simulink model "sm_boom_lift_crawler_test_jib_hydr_3D"  (R2026a)
settings: Solver=ode23t  StopTime=tVec.StopTime  MaxStep=2  AbsTol=1e-3
PostLoadFcn:
  | sm_boom_lift_crawler_settest('jib test')
StartFcn:
  | tic;
StopFcn:
  | Elapsed_Sim_Time = toc;
  | %disp(['Elapsed Sim Time = ' num2str(Elapsed_Sim_Time)]);
undefined symbols (not defined in the file): motion, oVec, tVec, X, Y, Z
libraries: nesl_utility x5, sm_lib x5, sm_boom_lift_crawler_lib x4, fl_lib x2, sm_boom_lift_crawler_lib_boom x1, sm_boom_lift_crawler_lib_actuators x1, sm_boom_lift_crawler_lib_inputs x1, simulink_extras x1
Description:
  | Copyright 2025-2026 The MathWorks, Inc.
settings Model: Creator=smiller  LastModifiedBy=smiller
settings SolverCC: MaxConsecutiveMinStep=5
settings DataIOCC: SignalLoggingName=logsout_sm_boom_lift_crawler
settings SimscapeCC: SimscapeNominalValues="[{\"value\":\"1\",\"unit\":\"A\"},{\"value\":\"nomval_psi\",\"unit\":\"psi\"},{\"value\":\"1\",\"unit\":\"cm^2\"},{\"value\":\"nomval_cmv3_s\",\"unit\":\"cm^3/s\"},{\"value\":\"1\",\"unit\":\"kJ/kg\"},{\"value\":\"1\",\"unit\":\"kW\"},{\"value\":\"1\",\"unit\":\"l\"},{\"value\":\"nomval_N\",\"unit\":\"N\"},{\"value\":\"nomval_Nm\",\"unit\":\"N*m\"},{\"value\":\"1\",\"unit\":\"V\"}]"  SimscapeLogName=simlog_sm_boom_lift_crawler  SimscapeLogLimitData=off  SimscapeLogDataHistory=5000.0
settings DiagnosticsConfigSet: SimMechanicsConflictingReferenceFrames=none  SimMechanicsRigidlyBoundBlock=none
settings ExplorerConfigSet: InternalSimMechanicsExplorerSettings="<ExplorerConfiguration><canonicalview>default</canonicalview><AnimationSetting><BasePlaybackSpeed>1.0</BasePlaybackSpeed><PlaybackSpeedFactor>8.0</PlaybackSpeedFactor></AnimationSetting><TilePanel><TileInfo><Tiles Columns=\"1\" Count=\"1\" Rows=\"1\"><Column Weight=\"1\"/><Row Weight=\"1\"/><Tile Height=\"1\" Width=\"1\" X=\"0\" Y=\"0\"/></Tiles></TileInfo><SceneInfo><SceneViewer><BGColor><R>1</R><G>1</G><B>1</B></BGColor><Camera><DoPerspective>on</DoPerspective><Position><X>3</X><Y>-0.999366517742438232</Y><Z>-0.50126496308374946</Z></Position><Center><X>2</X><Y>-0.999366517742438343</Y><Z>-0.501264963083749349</Z></Center><Up><X>0</X><Y>0</Y><Z>1</Z></Up><ViewLimDist>1</ViewLimDist><YLim>0.466307658154998583</YLim><XLim>0.785360266366313398</XLim></Camera></SceneViewer></SceneInfo></TilePanel><MechEditorPanel><Cameras><Camera><Id>Camera10</Id><Value><Name>Basket_Rotate</Name><NativeCamera><PositionTrackingFeature>Basket.Basket_Rotate.Bracket.Reference_Camera_Basket_Rotate_L.R</PositionTrackingFeature><CenterTrackingFeature>Basket.Basket_Rotate.Bracket.Reference_Camera_Basket_Rotate_L.R</CenterTrackingFeature><UpVectorTrackingFeature>Basket.Basket_Rotate.Bracket.Reference_Camera_Basket_Rotate_L.R</UpVectorTrackingFeature><CenterTrackingOrigin>off</CenterTrackingOrigin><CenterTrackingDirection>-X</CenterTrackingDirection><UpVectorTrackingDirection>+Z</UpVectorTrackingDirection></NativeCamera></Value></Camera><Camera><Id>Camera13</Id><Value><Name>View_Basket_World</Name><NativeCamera><PositionTrackingFeature>Basket.Basket.Reference_Basket_Cam.R</PositionTrackingFeature><CenterTrackingFeature>Mech_Config.World.W</CenterTrackingFeature><UpVectorTrackingFeature>Basket.Basket.Reference_Basket_Cam.R</UpVectorTrackingFeature><CenterTrackingOrigin>on</CenterTrackingOrigin><UpVectorTrackingDirection>+Y</UpVectorTrackingDirection></NativeCamera></Value></Camera><Camera><Id>Camera17</Id><Value><Name>Jib</Name><NativeCamera><PositionTrackingFeature>Basket.Jib.Jib_Mount.Reference_Camera_Basket_Jib.R</PositionTrackingFeature><CenterTrackingFeature>Basket.Jib.Jib_Mount.Reference_Camera_Basket_Jib.R</CenterTrackingFeature><UpVectorTrackingFeature>Mech_Config.World.W</UpVectorTrackingFeature><CenterTrackingOrigin>off</CenterTrackingOrigin><CenterTrackingDirection>-X</CenterTrackingDirection><UpVectorTrackingDirection>+Z</UpVectorTrackingDirection></NativeCamera></Value></Camera></Cameras><GfxPanelCameraMap><MapElement CameraMLId=\"Camera17\" GfxPanelIndex=\"0\"/></GfxPanelCameraMap><VideoCreator><PlaybackSpeedRatio>8</PlaybackSpeedRatio><FrameRate>30</FrameRate><VideoFormat>MPEG-4</VideoFormat><FrameSize>auto</FrameSize></VideoCreator></MechEditorPanel></ExplorerConfiguration>"

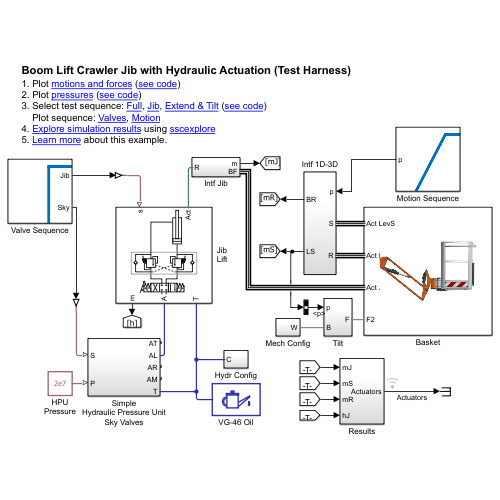
[thumbnail: Simulink's stored preview of the top-level diagram]
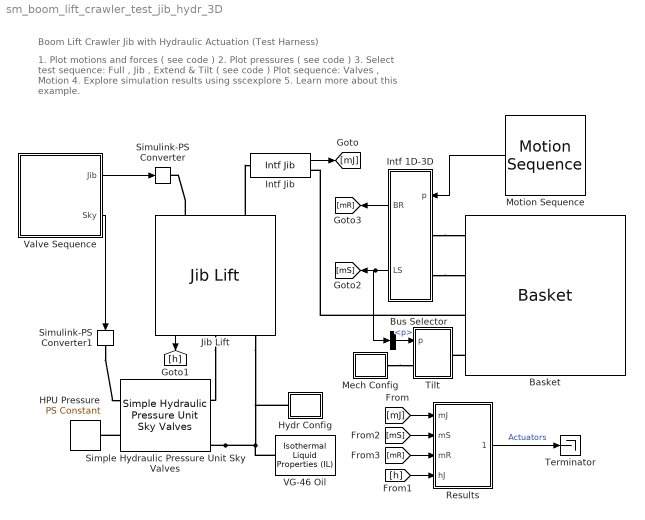
== system sm_boom_lift_crawler_test_jib_hydr_3D ==
  note: 1. Plot motions and forces ( see code )
      | 2. Plot pressures ( see code )
      | 3. Select test sequence: Full , Jib , Extend & Tilt ( see code )
      | Plot sequence: Valves , Motion
      | 4. Explore simulation results using sscexplore
      | 5. Learn more about this example.
  note: Boom Lift Crawler Jib with Hydraulic Actuation (Test Harness)
  Basket : sm_boom_lift_crawler_lib_boom/Boom/Basket  SystemSampleTime=-1  VariantActivationTime=update diagram  EmptyChoice=off  PassThrough=off  PassThroughVariantControl=(default)  EmptyChoiceVariantControl=(default)  AllowFlexibleInterface=on  Latency=0  AutoFrameSizeCalculation=off
  Bus Selector : BusSelector  OutputSignals=p
  HPU Pressure : fl_lib/Physical Signals/Sources/PS Constant  constant=2e7 Pa
  Hydr Config : Subsystem
  Intf 1D-3D : Subsystem
  Intf Jib : sm_boom_lift_crawler_lib/Intf Jib  SystemSampleTime=-1  VariantActivationTime=update diagram  EmptyChoice=off  PassThrough=off  PassThroughVariantControl=(default)  EmptyChoiceVariantControl=(default)  AllowFlexibleInterface=on  Latency=0  AutoFrameSizeCalculation=off
  Jib Lift : sm_boom_lift_crawler_lib_actuators/Actuators/Sky Manifold/Sky Valves II/Jib Lift  SystemSampleTime=-1  VariantActivationTime=update diagram  EmptyChoice=off  PassThrough=off  PassThroughVariantControl=(default)  EmptyChoiceVariantControl=(default)  AllowFlexibleInterface=on  Latency=0  AutoFrameSizeCalculation=off
  Mech Config : Subsystem
  Motion Sequence : sm_boom_lift_crawler_lib_inputs/Motion Sequence  SystemSampleTime=-1  VariantActivationTime=update diagram  EmptyChoice=off  PassThrough=off  PassThroughVariantControl=(default)  EmptyChoiceVariantControl=(default)  AllowFlexibleInterface=on  Latency=0  AutoFrameSizeCalculation=off
  Results : Subsystem
  Simple Hydraulic Pressure Unit Sky Valves : sm_boom_lift_crawler_lib/Simple Hydraulic Pressure Unit Sky Valves  SystemSampleTime=-1  VariantActivationTime=update diagram  EmptyChoice=off  PassThrough=off  PassThroughVariantControl=(default)  EmptyChoiceVariantControl=(default)  AllowFlexibleInterface=on  Latency=0  AutoFrameSizeCalculation=off
  Simulink-PS Converter : nesl_utility/Simulink-PS Converter  PhysicalDomain=network_engine_domain  SubClassName=ps_input  LeftPortType=input  RightPortType=output  PseudoPeriodic=off  Frequencies=[]  NoiseDistribution=none  NoiseParameters=[]  Unit=1  AffineConversion=off  FilteringAndDerivatives=provide  SimscapeFilterOrder=1  InputFilterTimeConstant=0.001  UdotUserProvided=0
  Simulink-PS Converter1 : nesl_utility/Simulink-PS Converter  PhysicalDomain=network_engine_domain  SubClassName=ps_input  LeftPortType=input  RightPortType=output  PseudoPeriodic=off  Frequencies=[]  NoiseDistribution=none  NoiseParameters=[]  Unit=1  AffineConversion=off  FilteringAndDerivatives=provide  SimscapeFilterOrder=1  InputFilterTimeConstant=0.001  UdotUserProvided=0
  Terminator : Terminator
  Tilt : Subsystem
  VG-46 Oil : fl_lib/Isothermal Liquid/Utilities/Isothermal Liquid Properties (IL)  rho_L_atm=867.346 kg/m^3  bulk_modulus_model=foundation.enum.bulk_modulus_model.const  beta_gain=6  beta_L_atm=1.48150e+09 Pa  nu_atm=(45.7333)*(1) cSt  p_atm=0.101325 MPa  p_min=1 Pa  properties_range_check=simscape.enum.assert.action.error  air_fraction=ratio_dissolved_air  polytropic_index=1.0  rho_g_atm=1.225 kg/m^3  air_dissolution_model=simscape.enum.onoff.off  p_crit=3 MPa
  Valve Sequence : Subsystem
      mask Display: image('sm_boom_lift_crawler_valve_seq_outputonly.svg');
  wires:
  Motion Sequence/1 -> Intf 1D-3D/1(p)
  Valve Sequence/2(Sky) -> Simulink-PS Converter1/1
  Intf 1D-3D/1(BR) -> [mR]
  [mR] -> Results/3(mR)
  Bus Selector/1 -> Tilt/1(p)  "<p>"
  [h] -> Results/4(hJ)
  Intf 1D-3D/2(LS) -> Bus Selector/1, [mS]
  Results/1(Actuators) -> Terminator/1  "Actuators"
  [mJ] -> Results/1(mJ)
  [mS] -> Results/2(mS)
  Intf Jib/1 -> [mJ]
  Jib Lift/1 -> [h]
  Valve Sequence/1(Jib) -> Simulink-PS Converter/1
  connections:
  Simple Hydraulic Pressure Unit Sky Valves/RConn5 -- Hydr Config/RConn1 -- Jib Lift/RConn2 -- VG-46 Oil/RConn1
  Basket/RConn3 -- Intf Jib/RConn1
  Mech Config/LConn1 -- Tilt/LConn1
  Simulink-PS Converter1/RConn1 -- Simple Hydraulic Pressure Unit Sky Valves/LConn1
  Intf 1D-3D/LConn1 -- Basket/RConn1
  Simple Hydraulic Pressure Unit Sky Valves/LConn2 -- HPU Pressure/RConn1
  Intf 1D-3D/LConn2 -- Basket/RConn2
  Jib Lift/LConn2 -- Intf Jib/LConn1
  Basket/RConn4 -- Tilt/RConn1
  Jib Lift/LConn1 -- Simulink-PS Converter/RConn1
  Jib Lift/RConn1 -- Simple Hydraulic Pressure Unit Sky Valves/RConn2

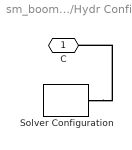
== system sm_boom_lift_crawler_test_jib_hydr_3D/Hydr Config ==
  Solver Configuration : nesl_utility/Solver Configuration  PhysicalDomain=network_engine_domain  SubClassName=solver  LeftPortType=input  RightPortType=generic  Tones=[]  Harmonics=[]  SimulateNoise=off  Profile=off  UseLocalSampling=off  EnableSwitchedLinearOptims=on  FrequencyDomain=off  UseCCode=off  RelTol=0.001  AbsTol=1e-06  MinStep=1e-09  ToWorkspace=off  RevertToSquareIcSolve=off  NumHomotopyIterations=100  PhasorMode=off  PhasorModeNumHarmonics=1  ConsistencySolver=NEWTON_FTOL  CanonicalOrdering=UNORDERED  OptimizeIntermediates=UNOPTIMIZED  IndexReductionMethod=DerivativeReplacement  DoDC=off  ResidualTolerance=1e-9  ConsistencyTolSource=GLOBAL  ConsistencyAbsTol=0.001  ConsistencyRelTol=0.001  ConsistencyTolFactor=0.001  UseLocalSolver=off  LocalSolverChoice=NE_BACKWARD_EULER_ADVANCER  ResolveIndetEquations=on  FunctionEvalNumThread=1  LocalSolverSampleTime=2e-3  DoFixedCost=off  MaxNonlinIter=5  MaxModeIter=2  ComputeImpulses=off  ImpulseIterations=2  LinearAlgebra=Sparse  LinearAlgebraNumThread=0  EquationFormulation=NE_TIME_EF  DelaysMemoryBudget=1024  AutomaticFiltering=on  FilteringTimeConstant=1e-3  PartitionStorageMethod=EXHAUSTIVE  PartitionMemoryBudget=1024  PartitionMethod=FAST  MultibodyUseLocalSolver=off  MultibodyLocalSolverChoice=ODE1  MultibodyLocalSolverSampleTime=0.001
  C : PMIOPort  Side=Right
  connections:
  Solver Configuration/RConn1 -- C/RConn1

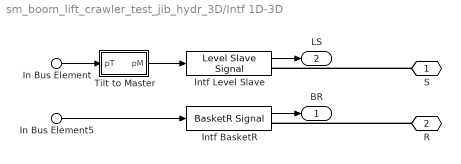
== system sm_boom_lift_crawler_test_jib_hydr_3D/Intf 1D-3D ==
  In Bus Element5 : Inport  PortName=p  Element=BasketR
  In Bus Element : Inport  PortName=p  Element=Tilt
  Intf BasketR : sm_boom_lift_crawler_lib/BasketR Signal  SystemSampleTime=-1  VariantActivationTime=update diagram  EmptyChoice=off  PassThrough=off  PassThroughVariantControl=(default)  EmptyChoiceVariantControl=(default)  AllowFlexibleInterface=on  Latency=0  AutoFrameSizeCalculation=off
  Intf Level Slave : sm_boom_lift_crawler_lib/Level Slave Signal  SystemSampleTime=-1  VariantActivationTime=update diagram  EmptyChoice=off  PassThrough=off  PassThroughVariantControl=(default)  EmptyChoiceVariantControl=(default)  AllowFlexibleInterface=on  Latency=0  AutoFrameSizeCalculation=off
  Tilt to Master : Subsystem
  S : PMIOPort  Side=Left
  R : PMIOPort  Port=2  Side=Left
  BR : Outport
  LS : Outport  Port=2
  wires:
  Intf Level Slave/1 -> LS/1
  Intf BasketR/1 -> BR/1
  In Bus Element5/1 -> Intf BasketR/1
  In Bus Element/1 -> Tilt to Master/1(pT)
  Tilt to Master/1(pM) -> Intf Level Slave/1
  connections:
  S/RConn1 -- Intf Level Slave/RConn1
  R/RConn1 -- Intf BasketR/RConn1

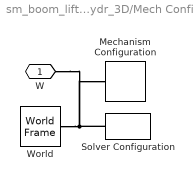
== system sm_boom_lift_crawler_test_jib_hydr_3D/Mech Config ==
  Mechanism Configuration : sm_lib/Utilities/Mechanism Configuration  UniformGravity=Constant  GravityVector=[0 0 -9.80665]  GravityVectorUnits=m/s^2  LinearizationDelta=0.001  JointModeTransitionNonlinearIterations=2
  Solver Configuration : nesl_utility/Solver Configuration  PhysicalDomain=network_engine_domain  SubClassName=solver  LeftPortType=input  RightPortType=generic  Tones=[]  Harmonics=[]  SimulateNoise=off  Profile=off  UseLocalSampling=off  EnableSwitchedLinearOptims=on  FrequencyDomain=off  UseCCode=off  RelTol=0.001  AbsTol=1e-06  MinStep=1e-09  ToWorkspace=off  RevertToSquareIcSolve=off  NumHomotopyIterations=100  PhasorMode=off  PhasorModeNumHarmonics=1  ConsistencySolver=NEWTON_FTOL  CanonicalOrdering=UNORDERED  OptimizeIntermediates=UNOPTIMIZED  IndexReductionMethod=DerivativeReplacement  DoDC=off  ResidualTolerance=1e-9  ConsistencyTolSource=GLOBAL  ConsistencyAbsTol=0.001  ConsistencyRelTol=0.001  ConsistencyTolFactor=0.001  UseLocalSolver=off  LocalSolverChoice=NE_BACKWARD_EULER_ADVANCER  ResolveIndetEquations=on  FunctionEvalNumThread=1  LocalSolverSampleTime=2e-3  DoFixedCost=off  MaxNonlinIter=3  MaxModeIter=2  ComputeImpulses=off  ImpulseIterations=2  LinearAlgebra=auto  LinearAlgebraNumThread=0  EquationFormulation=NE_TIME_EF  DelaysMemoryBudget=1024  AutomaticFiltering=on  FilteringTimeConstant=0.001  PartitionStorageMethod=AS_NEEDED  PartitionMemoryBudget=1024  PartitionMethod=ROBUST  MultibodyUseLocalSolver=off  MultibodyLocalSolverChoice=ODE1  MultibodyLocalSolverSampleTime=0.001
  World : sm_lib/Frames and Transforms/World Frame
  W : PMIOPort  Side=Left
  connections:
  Solver Configuration/RConn1 -- W/RConn1 -- Mechanism Configuration/RConn1 -- World/RConn1

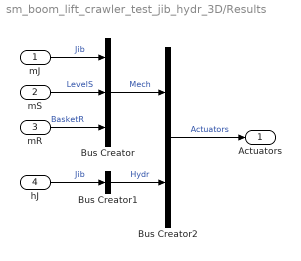
== system sm_boom_lift_crawler_test_jib_hydr_3D/Results ==
  mJ : Inport
  mS : Inport  Port=2
  mR : Inport  Port=3
  hJ : Inport  Port=4
  Bus Creator : BusCreator  Inputs=3
  Bus Creator1 : BusCreator  Inputs=1
  Bus Creator2 : BusCreator  Inputs=2
  Actuators : Outport
  wires:
  Bus Creator/1 -> Bus Creator2/1  "Mech"
  Bus Creator1/1 -> Bus Creator2/2  "Hydr"
  hJ/1 -> Bus Creator1/1  "Jib"
  mJ/1 -> Bus Creator/1  "Jib"
  Bus Creator2/1 -> Actuators/1  "Actuators"
  mS/1 -> Bus Creator/2  "LevelS"
  mR/1 -> Bus Creator/3  "BasketR"

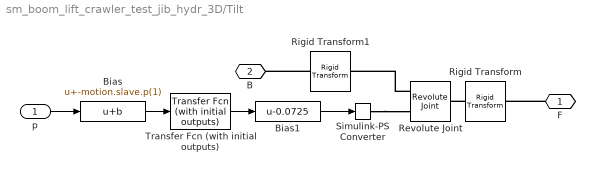
== system sm_boom_lift_crawler_test_jib_hydr_3D/Tilt ==
  p : Inport
  Bias : Bias  Bias=-motion.slave.p(1)  SaturateOnIntegerOverflow=off
  Bias1 : Bias  Bias=-0.0725  SaturateOnIntegerOverflow=off
  Revolute Joint : sm_lib/Joints/Revolute Joint  JointMode=Normal  CompositeWrenchDir=FollowerOnBase  CompositeWrenchFrame=BaseFrame  SenseConstraintForce=off  SenseConstraintTorque=off  SenseTotalForce=off  SenseTotalTorque=off  PositionTargetSpecify=on  PositionTargetPriority=High  PositionTargetValue=-0.0725  PositionTargetValueUnits=deg  VelocityTargetSpecify=off  VelocityTargetPriority=High  VelocityTargetValue=0  VelocityTargetValueUnits=deg/s  EquilibriumPosition=0  EquilibriumPositionUnits=deg  SpringStiffness=0  SpringStiffnessUnits=N*m/deg  DampingCoefficient=0  DampingCoefficientUnits=N*m/(deg/s)  LowerLimitSpecify=off  LowerLimitBound=-90  LowerLimitBoundUnits=deg  LowerLimitStiffness=1e4  LowerLimitStiffnessUnits=N*m/deg  LowerLimitDamping=10  LowerLimitDampingUnits=N*m/(deg/s)  LowerLimitTransitionRegionWidth=0.1  LowerLimitTransitionRegionWidthUnits=deg  UpperLimitSpecify=off  UpperLimitBound=90  UpperLimitBoundUnits=deg  UpperLimitStiffness=1e4  UpperLimitStiffnessUnits=N*m/deg  UpperLimitDamping=10  UpperLimitDampingUnits=N*m/(deg/s)  UpperLimitTransitionRegionWidth=0.1  UpperLimitTransitionRegionWidthUnits=deg  TorqueActuationMode=ComputedTorque  MotionActuationMode=InputMotion  SensePosition=off  SenseVelocity=off  SenseAcceleration=off  SenseTorqueForce=off  SenseLowerLimitTorqueForce=off  SenseUpperLimitTorqueForce=off
  Rigid Transform : sm_lib/Frames and Transforms/Rigid Transform  RotationMethod=StandardAxis  FollAlignAxisA=+X  BaseAlignAxisA=+Y  FollAlignAxisB=+Y  BaseAlignAxisB=+Z  RotationStandardAxis=+Y  RotationAngle=90  RotationAngleUnits=deg  RotationArbitraryAxis=[0 0 1]  RotationSequenceAxes=FollowerAxes  RotationSequence=XYX  RotationSequenceAngles=[0 0 0]  RotationSequenceAnglesUnits=deg  RotationMatrix=[1 0 0; 0 1 0; 0 0 1]  Quaternion=[1 0 0 0]  TranslationMethod=None  TranslationCartesianOffset=[0 0 0]  TranslationCartesianOffsetUnits=m  TranslationStandardAxis=+Z  TranslationStandardOffset=0  TranslationStandardOffsetUnits=m  TranslationROffset=0  TranslationROffsetUnits=m  TranslationThetaOffset=0  TranslationThetaOffsetUnits=deg  TranslationZOffset=0  TranslationZOffsetUnits=m
  Rigid Transform1 : sm_lib/Frames and Transforms/Rigid Transform  RotationMethod=StandardAxis  FollAlignAxisA=+X  BaseAlignAxisA=+Y  FollAlignAxisB=+Y  BaseAlignAxisB=+Z  RotationStandardAxis=+Y  RotationAngle=-90  RotationAngleUnits=deg  RotationArbitraryAxis=[0 0 1]  RotationSequenceAxes=FollowerAxes  RotationSequence=XYX  RotationSequenceAngles=[0 0 0]  RotationSequenceAnglesUnits=deg  RotationMatrix=[1 0 0; 0 1 0; 0 0 1]  Quaternion=[1 0 0 0]  TranslationMethod=None  TranslationCartesianOffset=[0 0 0]  TranslationCartesianOffsetUnits=m  TranslationStandardAxis=+Z  TranslationStandardOffset=0  TranslationStandardOffsetUnits=m  TranslationROffset=0  TranslationROffsetUnits=m  TranslationThetaOffset=0  TranslationThetaOffsetUnits=deg  TranslationZOffset=0  TranslationZOffsetUnits=m
  Simulink-PS Converter : nesl_utility/Simulink-PS Converter  PhysicalDomain=network_engine_domain  SubClassName=ps_input  LeftPortType=input  RightPortType=output  PseudoPeriodic=off  Frequencies=[]  NoiseDistribution=none  NoiseParameters=[]  Unit=deg  AffineConversion=off  FilteringAndDerivatives=filter  SimscapeFilterOrder=2  InputFilterTimeConstant=0.1  UdotUserProvided=0
  Transfer Fcn (with initial outputs) : simulink_extras/Additional Linear/Transfer Fcn (with initial outputs)  N=[400]  D="[0.1  1]"  Y0=0  U0=0
  F : PMIOPort  Side=Right
  B : PMIOPort  Port=2  Side=Left
  wires:
  Transfer Fcn (with initial outputs)/1 -> Bias1/1
  p/1 -> Bias/1
  Bias/1 -> Transfer Fcn (with initial outputs)/1
  Bias1/1 -> Simulink-PS Converter/1
  connections:
  F/RConn1 -- Rigid Transform/RConn1
  Revolute Joint/LConn1 -- Rigid Transform1/RConn1
  Rigid Transform1/LConn1 -- B/RConn1
  Rigid Transform/LConn1 -- Revolute Joint/RConn1
  Simulink-PS Converter/RConn1 -- Revolute Joint/LConn2

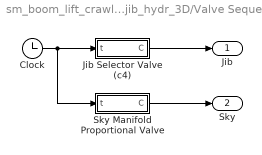
== system sm_boom_lift_crawler_test_jib_hydr_3D/Valve Sequence ==
  Clock : Clock
  Jib Selector Valve (c4) : Subsystem
  Sky Manifold Proportional Valve : Subsystem
  Jib : Outport
  Sky : Outport  Port=2
  wires:
  Sky Manifold Proportional Valve/1(C) -> Sky/1
  Clock/1 -> Jib Selector Valve (c4)/1(t), Sky Manifold Proportional Valve/1(t)
  Jib Selector Valve (c4)/1(C) -> Jib/1

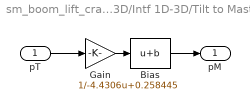
== system sm_boom_lift_crawler_test_jib_hydr_3D/Intf 1D-3D/Tilt to Master ==
  pT : Inport
  Bias : Bias  Bias=0.258445  SaturateOnIntegerOverflow=off
  Gain : Gain  Gain=1/-4.4306
  pM : Outport
  wires:
  Gain/1 -> Bias/1
  pT/1 -> Gain/1
  Bias/1 -> pM/1

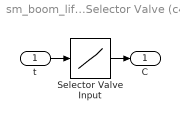
== system sm_boom_lift_crawler_test_jib_hydr_3D/Valve Sequence/Jib Selector Valve (c4) ==
  t : Inport
  Selector Valve Input : Lookup_n-D  NumberOfTableDimensions=1  BreakpointsForDimension1=tVec.sky.c4.all  Table=oVec.sky.c4.all  InterpMethod=Flat  ExtrapMethod=Clip  UseLastTableValue=on  InternalRulePriority=Speed  RndMeth=Simplest
  C : Outport
  wires:
  Selector Valve Input/1 -> C/1
  t/1 -> Selector Valve Input/1

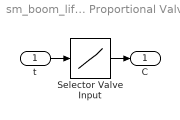
== system sm_boom_lift_crawler_test_jib_hydr_3D/Valve Sequence/Sky Manifold Proportional Valve ==
  t : Inport
  Selector Valve Input : Lookup_n-D  NumberOfTableDimensions=1  BreakpointsForDimension1=tVec.sky.proportional  Table=oVec.sky.proportional  InterpMethod=Flat  ExtrapMethod=Clip  UseLastTableValue=on  InternalRulePriority=Speed  RndMeth=Simplest
  C : Outport
  wires:
  t/1 -> Selector Valve Input/1
  Selector Valve Input/1 -> C/1
